simulink model "simulacao_realimentacao_estado_observado_v2"  (Simulink 8.9)
settings: Solver=ode45  StartTime=0.0  StopTime=1500  RelTol=1e-3  EnableMultiTasking=on
undefined symbols (not defined in the file): A, B, C, h3, K, Ki, L
libraries: simulink x2
settings Model: SuppressorTable=22 serialization::archive 11 0 6 0 0 0 11 0  Creator=admin  LastModifiedBy=root
settings OptimizationCC: ExpressionDepthLimit=2147483647
settings DebuggingCC: SolverPrmCheckMsg=warning

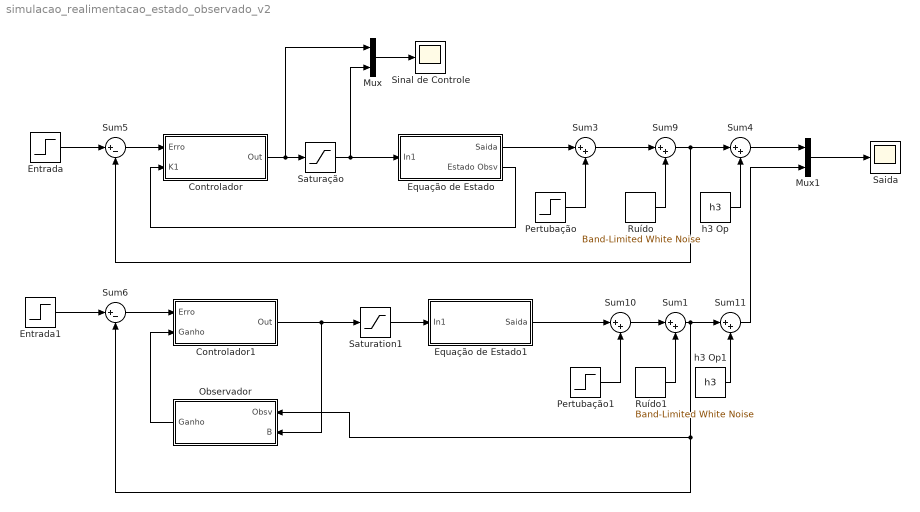
== system simulacao_realimentacao_estado_observado_v2 ==
  Controlador : Subsystem
  Controlador1 : Subsystem
  Entrada : Step  Time=0  SampleTime=0
  Entrada1 : Step  Time=0  SampleTime=0
  Equação de Estado : Subsystem
  Equação de Estado1 : Subsystem
  Mux : Mux  Inputs=2
  Mux1 : Mux  Inputs=2
  Observador : Subsystem
  Pertubação : Step  Time=1000  After=0.2  SampleTime=0
  Pertubação1 : Step  Time=1000  After=0.2  SampleTime=0
  Ruído : simulink/Sources/Band-Limited White Noise  Cov=[0.0001]  Ts=1  seed=[23341]
  Ruído1 : simulink/Sources/Band-Limited White Noise  Cov=[0.0001]  Ts=1  seed=[23341]
  Saida : Scope
  Saturation1 : Saturate  UpperLimit=4  LowerLimit=0
  Saturação : Saturate  UpperLimit=1  LowerLimit=0
  Sinal de Controle : Scope
  Sum{1,3..4,9..11} (6 alike) : Sum  Inputs=|++
  Sum5 : Sum  Inputs=|+-
  Sum6 : Sum  Inputs=|+-
  h3 Op : Constant  Value=h3
  h3 Op1 : Constant  Value=h3
  wires:
  Sum6/1 -> Controlador1/1(Erro)
  Controlador1/1(Out) -> Observador/2(B), Saturation1/1
  Entrada1/1 -> Sum6/1
  Saturação/1 -> Equação de Estado/1(In1), Mux/2
  Equação de Estado/2(Estado Obsv) -> Controlador/2(K1)
  Sum5/1 -> Controlador/1(Erro)
  Sum9/1 -> Sum5/2, Sum4/1
  Mux/1 -> Sinal de Controle/1
  Equação de Estado/1(Saida) -> Sum3/1
  Sum3/1 -> Sum9/1
  Pertubação/1 -> Sum3/2
  Entrada/1 -> Sum5/1
  Controlador/1(Out) -> Saturação/1, Mux/1
  h3 Op/1 -> Sum4/2
  Ruído/1 -> Sum9/2
  Sum4/1 -> Mux1/1
  Mux1/1 -> Saida/1
  Pertubação1/1 -> Sum10/2
  Equação de Estado1/1(Saida) -> Sum10/1
  Sum10/1 -> Sum1/1
  Ruído1/1 -> Sum1/2
  Sum1/1 -> Sum6/2, Observador/1(Obsv), Sum11/1
  h3 Op1/1 -> Sum11/2
  Sum11/1 -> Mux1/2
  Observador/1(Ganho) -> Controlador1/2(Ganho)
  Saturation1/1 -> Equação de Estado1/1(In1)

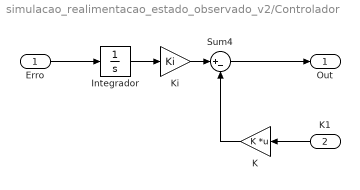
== system simulacao_realimentacao_estado_observado_v2/Controlador ==
  Erro : Inport
  K1 : Inport  Port=2
  Integrador : Integrator
  K : Gain  Gain=K  Multiplication=Matrix(K*u)
  Ki : Gain  Gain=Ki
  Sum4 : Sum  Inputs=|+-
  Out : Outport
  wires:
  K1/1 -> K/1
  Erro/1 -> Integrador/1
  Integrador/1 -> Ki/1
  K/1 -> Sum4/2
  Sum4/1 -> Out/1
  Ki/1 -> Sum4/1

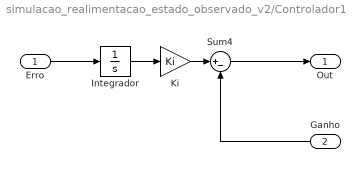
== system simulacao_realimentacao_estado_observado_v2/Controlador1 ==
  Erro : Inport
  Ganho : Inport  Port=2
  Integrador : Integrator
  Ki : Gain  Gain=Ki
  Sum4 : Sum  Inputs=|+-
  Out : Outport
  wires:
  Ki/1 -> Sum4/1
  Sum4/1 -> Out/1
  Integrador/1 -> Ki/1
  Erro/1 -> Integrador/1
  Ganho/1 -> Sum4/2

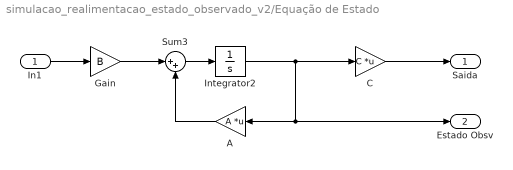
== system simulacao_realimentacao_estado_observado_v2/Equação de Estado ==
  In1 : Inport
  A : Gain  Gain=A  Multiplication=Matrix(K*u)
  C : Gain  Gain=C  Multiplication=Matrix(K*u)
  Gain : Gain  Gain=B
  Integrator2 : Integrator
  Sum3 : Sum  Inputs=|++
  Saida : Outport
  Estado Obsv : Outport  Port=2
  wires:
  Sum3/1 -> Integrator2/1
  Integrator2/1 -> C/1, A/1, Estado Obsv/1
  C/1 -> Saida/1
  A/1 -> Sum3/2
  Gain/1 -> Sum3/1
  In1/1 -> Gain/1

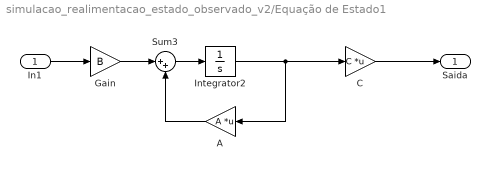
== system simulacao_realimentacao_estado_observado_v2/Equação de Estado1 ==
  In1 : Inport
  A : Gain  Gain=A  Multiplication=Matrix(K*u)
  C : Gain  Gain=C  Multiplication=Matrix(K*u)
  Gain : Gain  Gain=B
  Integrator2 : Integrator
  Sum3 : Sum  Inputs=|++
  Saida : Outport
  wires:
  A/1 -> Sum3/2
  C/1 -> Saida/1
  Integrator2/1 -> C/1, A/1
  Sum3/1 -> Integrator2/1
  In1/1 -> Gain/1
  Gain/1 -> Sum3/1

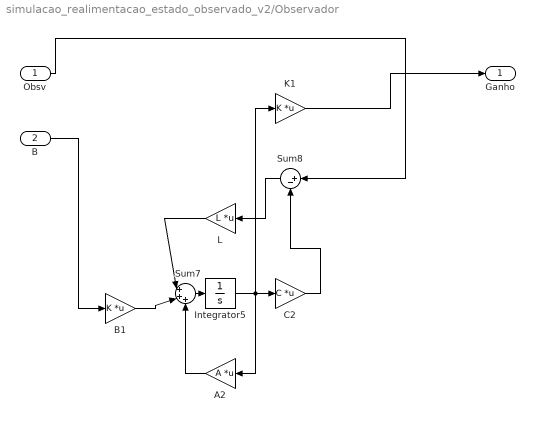
== system simulacao_realimentacao_estado_observado_v2/Observador ==
  Obsv : Inport
  B : Inport  Port=2
  A2 : Gain  Gain=A  Multiplication=Matrix(K*u)
  "B1 " : Gain  Gain=K  Multiplication=Matrix(K*u)
  C2 : Gain  Gain=C  Multiplication=Matrix(K*u)
  Integrator5 : Integrator
  K1 : Gain  Gain=K  Multiplication=Matrix(K*u)
  L : Gain  Gain=L  Multiplication=Matrix(K*u)
  Sum7 : Sum  Inputs=|+++
  Sum8 : Sum  Inputs=|+-
  Ganho : Outport
  wires:
  Integrator5/1 -> C2/1, A2/1, K1/1
  C2/1 -> Sum8/2
  Sum8/1 -> L/1
  L/1 -> Sum7/1
  "B1 "/1 -> Sum7/2
  A2/1 -> Sum7/3
  Sum7/1 -> Integrator5/1
  Obsv/1 -> Sum8/1
  K1/1 -> Ganho/1
  B/1 -> "B1 "/1
